simulink model "LQR_LE"  (R2024b)
settings: Solver=VariableStepAuto  StartTime=0.0  StopTime=10.0  RelTol=1e-3
values from neighbouring files (symbols this model uses):
  A = zeros(n)    [LinearizeHandle.m]
  B = (f(t0, x0, u0 + delta) - fx0u0) / delta    [LinearizeHandle.m]
  C = eye(n)    [LinearizeHandle.m]
  D = zeros(n, 1)    [LinearizeHandle.m]
  disorder_times = [10, 14]    [assignment1.m]
  lqr_stop_time = 15    [assignment1.m]
  u_control = 0.5    [assignment1.m]
  z = 0.1    [assignment1.m]
undefined symbols (not defined in the file or in its folder): K, N
settings Model: Creator=lukiq  LastModifiedBy=lukiq

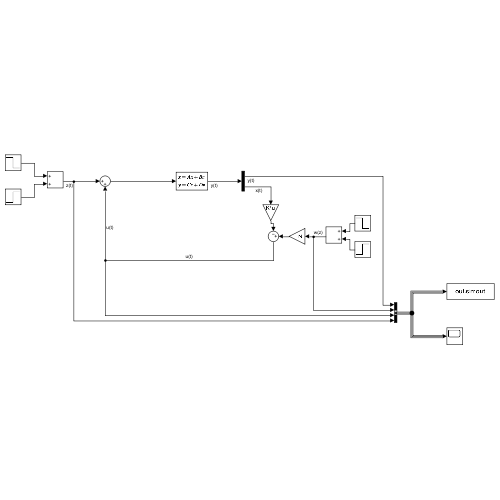
[thumbnail: Simulink's stored preview of the top-level diagram]
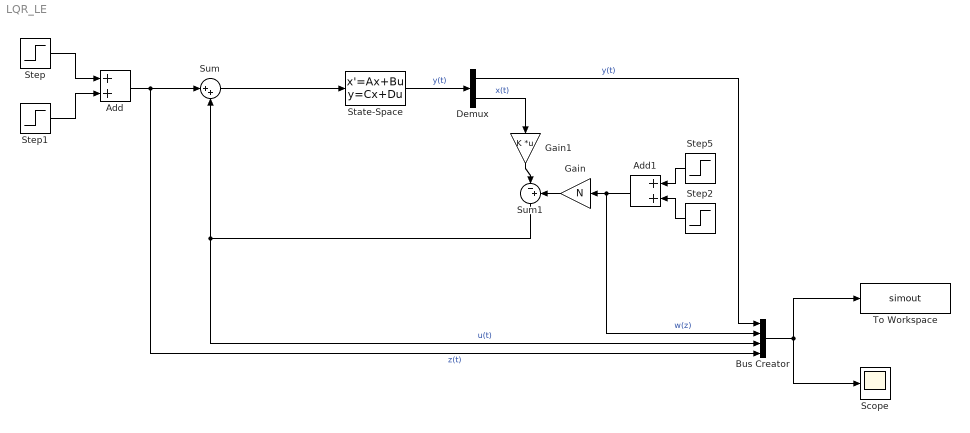
== system LQR_LE ==
  Add : Sum
  Add1 : Sum
  Bus Creator : BusCreator  Inputs=4
  Demux : Demux  Outputs=[1, 2]
  Gain : Gain  Gain=N
  Gain1 : Gain  Gain=K  Multiplication=Matrix(K*u)
  Scope : Scope
  State-Space : StateSpace  A=A  B=B  C=[C; eye(size(A))]  D=[D; zeros(size(B))]  InitialCondition=0
  Step : Step  Time=disorder_times(1)  After=- z * u_control  SampleTime=0
  Step1 : Step  Time=disorder_times(2)  After=z * u_control  SampleTime=0
  Step2 : Step  SampleTime=0
  Step5 : Step  Time=lqr_stop_time  After=-1  SampleTime=0
  Sum : Sum  Inputs=|++
  Sum1 : Sum  Inputs=|-+
  To Workspace : ToWorkspace  VariableName=simout  SaveFormat=Timeseries  SampleTime=-1
  wires:
  Sum/1 -> State-Space/1
  Sum1/1 -> Bus Creator/3, Sum/2  "u(t)"
  Add/1 -> Bus Creator/4, Sum/1  "z(t)"
  Step/1 -> Add/1
  Step1/1 -> Add/2
  Bus Creator/1 -> Scope/1, To Workspace/1
  Gain/1 -> Sum1/2
  Gain1/1 -> Sum1/1
  Step2/1 -> Add1/2
  Step5/1 -> Add1/1
  Add1/1 -> Bus Creator/2, Gain/1  "w(z)"
  State-Space/1 -> Demux/1  "y(t)"
  Demux/2 -> Gain1/1  "x(t)"
  Demux/1 -> Bus Creator/1  "y(t)"
